simulink subsystem "Direct_Roll_and_Pitch_Command"  (R2023a)
settings: Solver=VariableStepAuto  StartTime=0.0  StopTime=10.0  RelTol=1e-3
libraries: simulink x2, eeGeneralControl x2
settings Model: Creator=thesa  LastModifiedBy=thesa

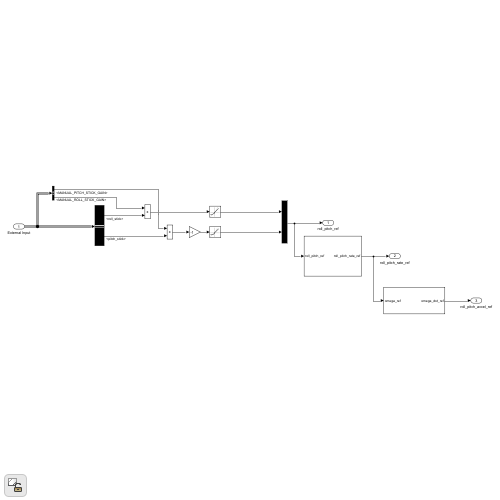
[thumbnail: Simulink's stored preview of the top-level diagram]
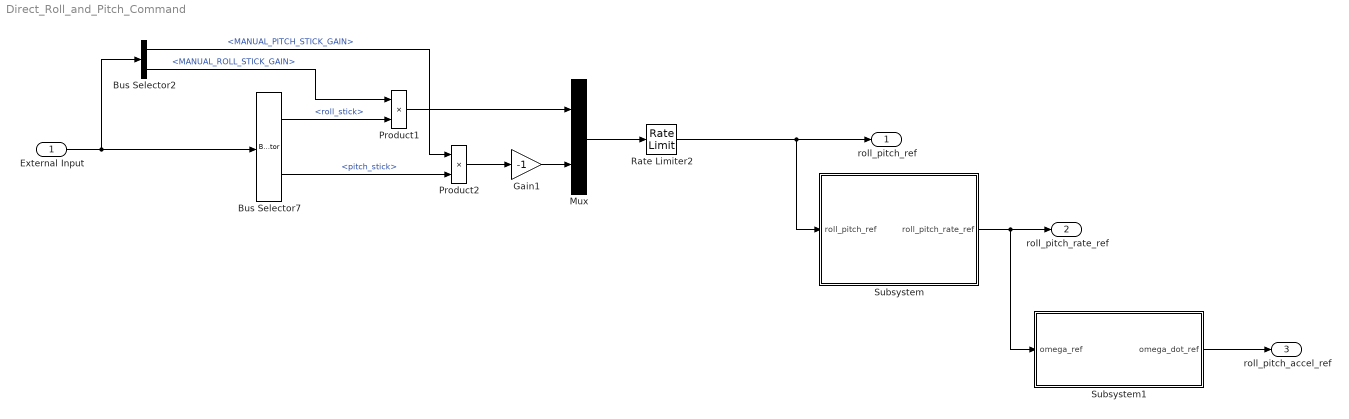
== system Direct_Roll_and_Pitch_Command ==
  External Input : Inport
  Bus Selector2 : BusSelector  OutputSignals=Pilot Input.Parameters.MANUAL_PITCH_STICK_GAIN,Pilot Input.Parameters.MANUAL_ROLL_STICK_GAIN
  Bus Selector7 : BusSelector  OutputSignals=Pilot Input.Sticks.roll_stick,Pilot Input.Sticks.pitch_stick
  Gain1 : Gain  Gain=-1
  Mux : Mux  Inputs=2
  Product1 : Product
  Product2 : Product
  Rate Limiter2 : RateLimiter  RisingSlewLimit=60*pi/180  FallingSlewLimit=-60*pi/180  SampleTimeMode=inherited
  Subsystem : Subsystem
  Subsystem1 : Subsystem
  roll_pitch_ref : Outport
  roll_pitch_rate_ref : Outport  Port=2
  roll_pitch_accel_ref : Outport  Port=3
  wires:
  Bus Selector7/2 -> Product2/2  "<pitch_stick>"
  Bus Selector7/1 -> Product1/2  "<roll_stick>"
  External Input/1 -> Bus Selector2/1, Bus Selector7/1
  Subsystem/1(roll_pitch_rate_ref) -> Subsystem1/1(omega_ref), roll_pitch_rate_ref/1
  Mux/1 -> Rate Limiter2/1
  Bus Selector2/2 -> Product1/1  "<MANUAL_ROLL_STICK_GAIN>"
  Bus Selector2/1 -> Product2/1  "<MANUAL_PITCH_STICK_GAIN>"
  Product2/1 -> Gain1/1
  Gain1/1 -> Mux/2
  Product1/1 -> Mux/1
  Subsystem1/1(omega_dot_ref) -> roll_pitch_accel_ref/1
  Rate Limiter2/1 -> roll_pitch_ref/1, Subsystem/1(roll_pitch_ref)

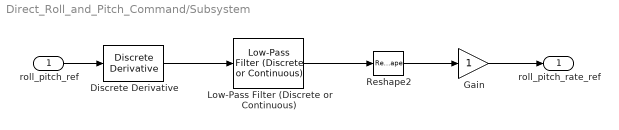
== system Direct_Roll_and_Pitch_Command/Subsystem ==
  roll_pitch_ref : Inport
  Discrete Derivative : simulink/Discrete/Discrete Derivative  gainval=1.0  ICPrevScaledInput=0.0  OutMin=[]  OutMax=[]  OutDataType=fixdt(1, 16)  OutScaling=2^-10  DoSatur=off
  Gain : Gain
  Low-Pass Filter (Discrete or Continuous) : eeGeneralControl/Low-Pass Filter (Discrete or Continuous)  K=1  T=1/20  B=inf  A=-inf  init_option=Inherited from block input  x0=0  Ts=-1
  Reshape2 : Reshape  OutputDimensionality=Column vector (2-D)
  roll_pitch_rate_ref : Outport
  wires:
  Reshape2/1 -> Gain/1
  Discrete Derivative/1 -> Low-Pass Filter (Discrete or Continuous)/1
  Low-Pass Filter (Discrete or Continuous)/1 -> Reshape2/1
  roll_pitch_ref/1 -> Discrete Derivative/1
  Gain/1 -> roll_pitch_rate_ref/1

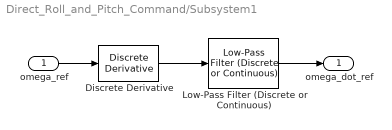
== system Direct_Roll_and_Pitch_Command/Subsystem1 ==
  omega_ref : Inport
  Discrete Derivative : simulink/Discrete/Discrete Derivative  gainval=1.0  ICPrevScaledInput=0.0  OutMin=[]  OutMax=[]  OutDataType=fixdt(1, 16)  OutScaling=2^-10  DoSatur=off
  Low-Pass Filter (Discrete or Continuous) : eeGeneralControl/Low-Pass Filter (Discrete or Continuous)  K=1  T=1/40  B=inf  A=-inf  init_option=Inherited from block input  x0=0  Ts=-1
  omega_dot_ref : Outport
  wires:
  Low-Pass Filter (Discrete or Continuous)/1 -> omega_dot_ref/1
  omega_ref/1 -> Discrete Derivative/1
  Discrete Derivative/1 -> Low-Pass Filter (Discrete or Continuous)/1
